simulink model "section_6_2_second_group"  (R2020a)
settings: Solver=ode45  StartTime=0.0  StopTime=50  RelTol=1e-5  EnableMultiTasking=on
(part 1 of 4)
settings Model: Creator=13018  LastModifiedBy=YW
settings DataIOCC: ReturnWorkspaceOutputs=off
settings OptimizationCC: LifeSpan=inf
settings DebuggingCC: SFUnexpectedBacktrackingDiag=warning  SFNoUnconditionalDefaultTransitionDiag=warning  ArithmeticOperatorsInVariantConditions=warning
settings SFSimCC: SimUseLocalCustomCode=off  CustomCodeUndefinedFunction=UseInterfaceOnly
settings RTWCC: RTWUseLocalCustomCode=off
settings CodeAppCC: StateflowObjectComments=on
settings GRTTargetCC: TargetLangStandard=C89/C90 (ANSI)
settings ConfigComp: CovMetricSettings=dw  CovHtmlReporting=on  CovSaveCumulativeToWorkspaceVar=on  CovSaveSingleToWorkspaceVar=on  CovExternalEMLEnable=off

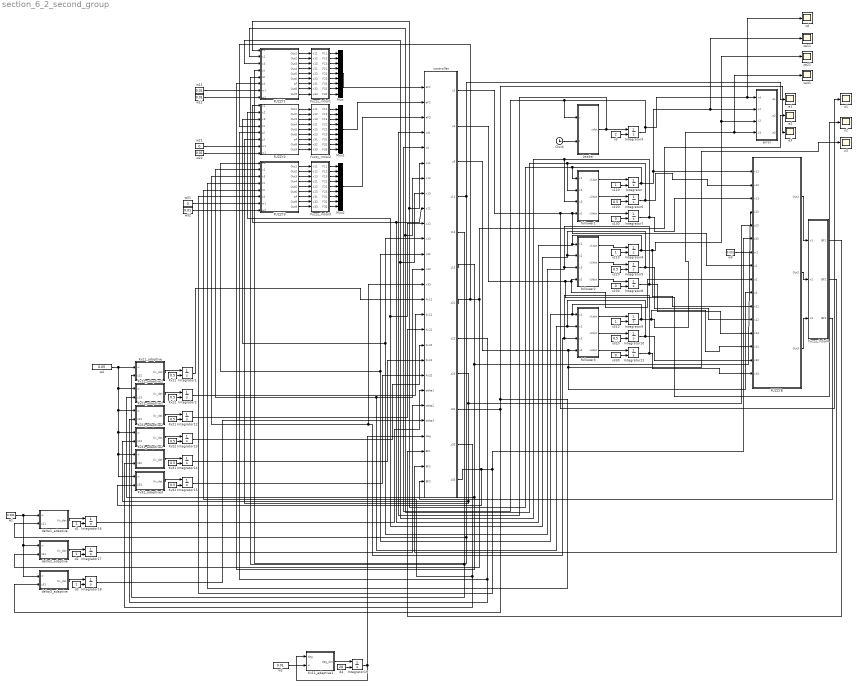
== system section_6_2_second_group ==
  Clock : Clock
  FUZZY1 : Subsystem
  FUZZY2 : Subsystem
  FUZZY3 : Subsystem
  FUZZYB : Subsystem
  Fuzzy_intial1 : MATLAB Function  TreatAsAtomicUnit=on
  Fuzzy_intial2 : MATLAB Function  TreatAsAtomicUnit=on
  Fuzzy_intial3 : MATLAB Function  TreatAsAtomicUnit=on
  Fuzzy_intial4 : MATLAB Function  TreatAsAtomicUnit=on
  Integrator{,1..19} (20 alike) : Integrator  InitialConditionSource=external
  Kv{11..12,21..22,31..32} (6 alike) : Constant  Value=0.5  VectorParams1D=off  SampleTime=-1
  Kv11_adaptive : MATLAB Function  TreatAsAtomicUnit=on
  Kv11_adaptive1 : MATLAB Function  TreatAsAtomicUnit=on
  Kv12_adaptive1 : MATLAB Function  TreatAsAtomicUnit=on
  Kv21_adaptive1 : MATLAB Function  TreatAsAtomicUnit=on
  Kv22_adaptive2 : MATLAB Function  TreatAsAtomicUnit=on
  Kv31_adaptive2 : MATLAB Function  TreatAsAtomicUnit=on
  Kv32_adaptive3 : MATLAB Function  TreatAsAtomicUnit=on
  Leader : MATLAB Function  TreatAsAtomicUnit=on
  Mux : Mux  Inputs=9
  Mux1 : Mux  Inputs=9
  Mux2 : Mux  Inputs=9
  controller : MATLAB Function  TreatAsAtomicUnit=on
  d1 : Constant  VectorParams1D=off  SampleTime=-1
  d2 : Constant  VectorParams1D=off  SampleTime=-1
  d3 : Constant  VectorParams1D=off  SampleTime=-1
  d4 : Constant  Value=20  VectorParams1D=off  SampleTime=-1
  delta1_adaptive : MATLAB Function  TreatAsAtomicUnit=on
  delta2_adaptive : MATLAB Function  TreatAsAtomicUnit=on
  delta3_adaptive : MATLAB Function  TreatAsAtomicUnit=on
  e1 : Scope
  e2 : Scope
  e3 : Scope
  error : MATLAB Function  TreatAsAtomicUnit=on
  follower1 : MATLAB Function  TreatAsAtomicUnit=on
  follower2 : MATLAB Function  TreatAsAtomicUnit=on
  follower3 : MATLAB Function  TreatAsAtomicUnit=on
  u1 : Scope
  u2 : Scope
  u3 : Scope
  w1 : Constant  Value=0.001  VectorParams1D=off  SampleTime=-1
  w{2,11..12,22,32} (5 alike) : Constant  Value=0.01  VectorParams1D=off  SampleTime=-1
  w21 : Constant  Value=0  VectorParams1D=off  SampleTime=-1
  w3 : Constant  Value=0.001  VectorParams1D=off  SampleTime=-1
  w31 : Constant  Value=0  VectorParams1D=off  SampleTime=-1
  w4 : Constant  Value=0.05  VectorParams1D=off  SampleTime=-1
  x0 : Constant  Value=2  VectorParams1D=off  SampleTime=-1
  x110 : Constant  VectorParams1D=off  SampleTime=-1
  x120 : Constant  Value=0.5  VectorParams1D=off  SampleTime=-1
  x130 : Constant  Value=0  VectorParams1D=off  SampleTime=-1
  x210 : Constant  VectorParams1D=off  SampleTime=-1
  x220 : Constant  Value=0.5  VectorParams1D=off  SampleTime=-1
  x230 : Constant  Value=0  VectorParams1D=off  SampleTime=-1
  x310 : Constant  VectorParams1D=off  SampleTime=-1
  x320 : Constant  Value=0.5  VectorParams1D=off  SampleTime=-1
  x330 : Constant  Value=0  VectorParams1D=off  SampleTime=-1
  xa11 : Scope
  xa21 : Scope
  xa31 : Scope
  xd : Scope
  wires:
  follower1/1(x1dot) -> Integrator/1
  Leader/1(xdot) -> controller/4(xdt), Integrator3/1
  x0/1 -> Integrator3/2
  follower1/2(x2dot) -> Integrator6/1
  follower1/3(x3dot) -> Integrator7/1
  x110/1 -> Integrator/2
  Integrator6/1 -> FUZZYB/2(x12), follower1/2(x2), FUZZY1/2(x2), controller/7(x12)
  Integrator7/1 -> FUZZYB/3(x13), FUZZY1/3(x3), controller/8(x13), follower1/3(x3)
  follower2/1(x1dot) -> Integrator4/1
  Integrator4/1 -> FUZZYB/11(x21), xa21/1, error/3(x2), FUZZY2/1(x1), controller/9(x21), follower2/1(x1)
  follower2/2(x2dot) -> Integrator5/1
  follower2/3(x3dot) -> Integrator8/1
  x210/1 -> Integrator4/2
  Integrator5/1 -> FUZZYB/12(x22), FUZZY2/2(x2), controller/10(x22), follower2/2(x2)
  Integrator8/1 -> FUZZYB/13(x23), FUZZY2/3(x3), controller/11(x23), follower2/3(x3)
  follower3/1(x1dot) -> Integrator9/1
  follower3/2(x2dot) -> Integrator10/1
  follower3/3(x3dot) -> Integrator11/1
  x310/1 -> Integrator9/2
  controller/1(u1) -> u1/1, FUZZYB/8(u1), follower1/4(u1)
  controller/2(u2) -> u2/1, FUZZYB/9(u2), follower2/4(u2)
  controller/3(u3) -> FUZZYB/10(u3), u3/1, follower3/4(u3)
  controller/5(z12) -> FUZZY1/5(z2), Kv11_adaptive/2(z12)
  controller/6(z13) -> FUZZYB/4(z13), FUZZY1/6(z3), Kv12_adaptive1/2(z13)
  controller/8(z22) -> FUZZY2/5(z2), Kv21_adaptive1/2(z22)
  controller/9(z23) -> FUZZYB/5(z23), FUZZY2/6(z3), Kv22_adaptive2/2(z23)
  controller/11(z32) -> FUZZY3/5(z2), Kv31_adaptive2/2(z32)
  controller/12(z33) -> FUZZYB/6(z33), FUZZY3/6(z3), Kv32_adaptive3/2(z33)
  Kv11_adaptive/1(Kv_dot) -> Integrator1/1
  Kv11/1 -> Integrator1/2
  Integrator1/1 -> controller/15(Kv11)
  Kv12_adaptive1/1(Kv_dot) -> Integrator2/1
  Kv12/1 -> Integrator2/2
  Kv21_adaptive1/1(Kv_dot) -> Integrator12/1
  Kv21/1 -> Integrator12/2
  Kv22_adaptive2/1(Kv_dot) -> Integrator13/1
  Kv22/1 -> Integrator13/2
  Kv31_adaptive2/1(Kv_dot) -> Integrator14/1
  Kv31/1 -> Integrator14/2
  Kv32_adaptive3/1(Kv_dot) -> Integrator15/1
  Kv32/1 -> Integrator15/2
  Integrator2/1 -> controller/16(Kv12)
  Integrator13/1 -> controller/18(Kv22)
  Integrator12/1 -> controller/17(Kv21)
  Integrator14/1 -> controller/19(Kv31)
  Integrator15/1 -> controller/20(Kv32)
  Clock/1 -> Leader/2(t)
  Mux/1 -> controller/1(aF1)
  Mux2/1 -> controller/3(aF3)
  Mux1/1 -> controller/2(aF2)
  w11/1 -> FUZZY1/7(w1)
  w12/1 -> FUZZY1/8(w2)
  w21/1 -> FUZZY2/7(w1)
  w22/1 -> FUZZY2/8(w2)
  w32/1 -> FUZZY3/8(w2)
  w31/1 -> FUZZY3/7(w1)
  delta1_adaptive/1(Kv_dot) -> Integrator16/1
  d1/1 -> Integrator16/2
  delta2_adaptive/1(Kv_dot) -> Integrator17/1
  d2/1 -> Integrator17/2
  delta3_adaptive/1(Kv_dot) -> Integrator18/1
  d3/1 -> Integrator18/2
  w1/1 -> delta3_adaptive/1(w), delta2_adaptive/1(w), delta1_adaptive/1(w)
  Integrator16/1 -> controller/21(delta1)
  Integrator17/1 -> controller/22(delta2)
  Integrator18/1 -> controller/23(delta3)
  FUZZY1/1(Out1) -> Fuzzy_intial1/1(x11)
  FUZZY1/2(Out2) -> Fuzzy_intial1/2(x12)
  FUZZY1/3(Out3) -> Fuzzy_intial1/3(x13)
  FUZZY1/4(Out4) -> Fuzzy_intial1/4(x21)
  FUZZY1/5(Out5) -> Fuzzy_intial1/5(x22)
  FUZZY1/6(Out6) -> Fuzzy_intial1/6(x23)
  FUZZY1/7(aF) -> Fuzzy_intial1/7(x31)
  FUZZY1/8(Out8) -> Fuzzy_intial1/8(x32)
  FUZZY1/9(Out9) -> Fuzzy_intial1/9(x33)
  Fuzzy_intial1/1(F11) -> Mux/1
  Fuzzy_intial1/2(F12) -> Mux/2
  Fuzzy_intial1/3(F13) -> Mux/3
  Fuzzy_intial1/4(F21) -> Mux/4
  Fuzzy_intial1/5(F22) -> Mux/5
  Fuzzy_intial1/6(F23) -> Mux/6
  Fuzzy_intial1/7(F31) -> Mux/7
  Fuzzy_intial1/8(F32) -> Mux/8
  Fuzzy_intial1/9(F33) -> Mux/9
  Fuzzy_intial2/1(F11) -> Mux1/1
  Fuzzy_intial2/2(F12) -> Mux1/2
  Fuzzy_intial2/3(F13) -> Mux1/3
  Fuzzy_intial2/4(F21) -> Mux1/4
  Fuzzy_intial2/5(F22) -> Mux1/5
  Fuzzy_intial2/6(F23) -> Mux1/6
  Fuzzy_intial2/7(F31) -> Mux1/7
  Fuzzy_intial2/8(F32) -> Mux1/8
  Fuzzy_intial2/9(F33) -> Mux1/9
  FUZZY2/1(Out1) -> Fuzzy_intial2/1(x11)
  FUZZY2/2(Out2) -> Fuzzy_intial2/2(x12)
  FUZZY2/3(Out3) -> Fuzzy_intial2/3(x13)
  FUZZY2/4(Out4) -> Fuzzy_intial2/4(x21)
  FUZZY2/5(Out5) -> Fuzzy_intial2/5(x22)
  FUZZY2/6(Out6) -> Fuzzy_intial2/6(x23)
  FUZZY2/7(aF) -> Fuzzy_intial2/7(x31)
  FUZZY2/8(Out8) -> Fuzzy_intial2/8(x32)
  FUZZY2/9(Out9) -> Fuzzy_intial2/9(x33)
  Fuzzy_intial3/1(F11) -> Mux2/1
  Fuzzy_intial3/2(F12) -> Mux2/2
  Fuzzy_intial3/3(F13) -> Mux2/3
  Fuzzy_intial3/4(F21) -> Mux2/4
  Fuzzy_intial3/5(F22) -> Mux2/5
  Fuzzy_intial3/6(F23) -> Mux2/6
  Fuzzy_intial3/7(F31) -> Mux2/7
  Fuzzy_intial3/8(F32) -> Mux2/8
  Fuzzy_intial3/9(F33) -> Mux2/9
  FUZZY3/1(Out1) -> Fuzzy_intial3/1(x11)
  FUZZY3/2(Out2) -> Fuzzy_intial3/2(x12)
  FUZZY3/3(Out3) -> Fuzzy_intial3/3(x13)
  FUZZY3/4(Out4) -> Fuzzy_intial3/4(x21)
  FUZZY3/5(Out5) -> Fuzzy_intial3/5(x22)
  FUZZY3/6(Out6) -> Fuzzy_intial3/6(x23)
  FUZZY3/7(aF) -> Fuzzy_intial3/7(x31)
  FUZZY3/8(Out8) -> Fuzzy_intial3/8(x32)
  FUZZY3/9(Out9) -> Fuzzy_intial3/9(x33)
  w4/1 -> Kv32_adaptive3/1(w), Kv31_adaptive2/1(w), Kv22_adaptive2/1(w), Kv21_adaptive1/1(w), Kv12_adaptive1/1(w), Kv11_adaptive/1(w)
  Kv11_adaptive1/1(dag_dot) -> Integrator19/1
  d4/1 -> Integrator19/2
  Integrator19/1 -> controller/24(dag), Kv11_adaptive1/1(dag)
  w2/1 -> Kv11_adaptive1/2(w)
  Integrator10/1 -> FUZZYB/15(x32), follower3/2(x2), FUZZY3/2(x2), controller/13(x32)
  Integrator11/1 -> FUZZYB/16(x33), FUZZY3/3(x3), controller/14(x33), follower3/3(x3)
  FUZZYB/1(Out1) -> Fuzzy_intial4/1(x1)
  FUZZYB/2(Out2) -> Fuzzy_intial4/2(x2)
  FUZZYB/3(Out3) -> Fuzzy_intial4/3(x3)
  Fuzzy_intial4/1(BF1) -> controller/25(BF1)
  Fuzzy_intial4/2(BF2) -> controller/26(BF2)
  Fuzzy_intial4/3(BF3) -> controller/27(BF3)
  w3/1 -> FUZZYB/7(w1)
  controller/4(z11) -> FUZZY1/4(z1), delta1_adaptive/2(z11), e1/1
  controller/7(z21) -> FUZZY2/4(z1), delta2_adaptive/2(z21), e2/1
  controller/10(z31) -> FUZZY3/4(z1), e3/1, delta3_adaptive/2(z31)
  x120/1 -> Integrator6/2
  x130/1 -> Integrator7/2
  x220/1 -> Integrator5/2
  x230/1 -> Integrator8/2
  x320/1 -> Integrator10/2
  x330/1 -> Integrator11/2
  Integrator3/1 -> xd/1, error/1(xd), Leader/1(x), controller/5(xd)
  Integrator/1 -> FUZZYB/1(x11), xa11/1, error/2(x1), follower1/1(x1), FUZZY1/1(x1), controller/6(x11)
  Integrator9/1 -> FUZZYB/14(x31), xa31/1, error/4(x3), FUZZY3/1(x1), controller/12(x31), follower3/1(x1)

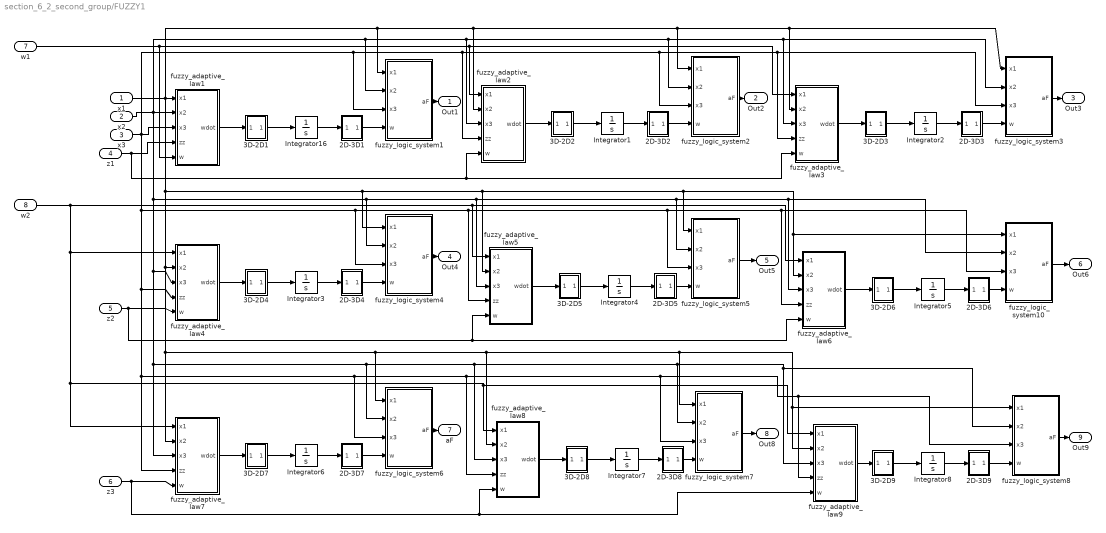
== system section_6_2_second_group/FUZZY1 ==
  x1 : Inport
  x2 : Inport  Port=2
  x3 : Inport  Port=3
  z1 : Inport  Port=4
  z2 : Inport  Port=5
  z3 : Inport  Port=6
  w1 : Inport  Port=7
  w2 : Inport  Port=8
  2D-3D1 : MATLAB Function  TreatAsAtomicUnit=on
  2D-3D2 : MATLAB Function  TreatAsAtomicUnit=on
  2D-3D3 : MATLAB Function  TreatAsAtomicUnit=on
  2D-3D4 : MATLAB Function  TreatAsAtomicUnit=on
  2D-3D5 : MATLAB Function  TreatAsAtomicUnit=on
  2D-3D6 : MATLAB Function  TreatAsAtomicUnit=on
  2D-3D7 : MATLAB Function  TreatAsAtomicUnit=on
  2D-3D8 : MATLAB Function  TreatAsAtomicUnit=on
  2D-3D9 : MATLAB Function  TreatAsAtomicUnit=on
  3D-2D1 : MATLAB Function  TreatAsAtomicUnit=on
  3D-2D2 : MATLAB Function  TreatAsAtomicUnit=on
  3D-2D3 : MATLAB Function  TreatAsAtomicUnit=on
  3D-2D4 : MATLAB Function  TreatAsAtomicUnit=on
  3D-2D5 : MATLAB Function  TreatAsAtomicUnit=on
  3D-2D6 : MATLAB Function  TreatAsAtomicUnit=on
  3D-2D7 : MATLAB Function  TreatAsAtomicUnit=on
  3D-2D8 : MATLAB Function  TreatAsAtomicUnit=on
  3D-2D9 : MATLAB Function  TreatAsAtomicUnit=on
  Integrator{1..8,16} (9 alike) : Integrator
  fuzzy_adaptive_law1 : MATLAB Function  TreatAsAtomicUnit=on
  fuzzy_adaptive_law2 : MATLAB Function  TreatAsAtomicUnit=on
  fuzzy_adaptive_law3 : MATLAB Function  TreatAsAtomicUnit=on
  fuzzy_adaptive_law4 : MATLAB Function  TreatAsAtomicUnit=on
  fuzzy_adaptive_law5 : MATLAB Function  TreatAsAtomicUnit=on
  fuzzy_adaptive_law6 : MATLAB Function  TreatAsAtomicUnit=on
  fuzzy_adaptive_law7 : MATLAB Function  TreatAsAtomicUnit=on
  fuzzy_adaptive_law8 : MATLAB Function  TreatAsAtomicUnit=on
  fuzzy_adaptive_law9 : MATLAB Function  TreatAsAtomicUnit=on
  fuzzy_logic_system1 : MATLAB Function  TreatAsAtomicUnit=on
  fuzzy_logic_system10 : MATLAB Function  TreatAsAtomicUnit=on
  fuzzy_logic_system2 : MATLAB Function  TreatAsAtomicUnit=on
  fuzzy_logic_system3 : MATLAB Function  TreatAsAtomicUnit=on
  fuzzy_logic_system4 : MATLAB Function  TreatAsAtomicUnit=on
  fuzzy_logic_system5 : MATLAB Function  TreatAsAtomicUnit=on
  fuzzy_logic_system6 : MATLAB Function  TreatAsAtomicUnit=on
  fuzzy_logic_system7 : MATLAB Function  TreatAsAtomicUnit=on
  fuzzy_logic_system8 : MATLAB Function  TreatAsAtomicUnit=on
  Out1 : Outport
  Out2 : Outport  Port=2
  Out3 : Outport  Port=3
  Out4 : Outport  Port=4
  Out5 : Outport  Port=5
  Out6 : Outport  Port=6
  aF : Outport  Port=7
  Out8 : Outport  Port=8
  Out9 : Outport  Port=9
  wires:
  3D-2D1/1(y) -> Integrator16/1
  fuzzy_adaptive_law1/1(wdot) -> 3D-2D1/1(x)
  Integrator16/1 -> 2D-3D1/1(x)
  2D-3D1/1(y) -> fuzzy_logic_system1/4(w)
  3D-2D2/1(y) -> Integrator1/1
  fuzzy_adaptive_law2/1(wdot) -> 3D-2D2/1(x)
  Integrator1/1 -> 2D-3D2/1(x)
  2D-3D2/1(y) -> fuzzy_logic_system2/4(w)
  3D-2D3/1(y) -> Integrator2/1
  fuzzy_adaptive_law3/1(wdot) -> 3D-2D3/1(x)
  Integrator2/1 -> 2D-3D3/1(x)
  2D-3D3/1(y) -> fuzzy_logic_system3/4(w)
  x1/1 -> fuzzy_adaptive_law4/2(x2), fuzzy_adaptive_law7/2(x2), fuzzy_logic_system6/1(x1), fuzzy_adaptive_law8/2(x2), fuzzy_adaptive_law9/2(x2), fuzzy_logic_system8/1(x1), fuzzy_logic_system7/1(x1), fuzzy_adaptive_law5/2(x2), fuzzy_logic_system5/1(x1), fuzzy_adaptive_law6/2(x2), fuzzy_logic_system10/1(x1), fuzzy_logic_system4/1(x1), fuzzy_adaptive_law1/1(x1), fuzzy_logic_system1/1(x1), fuzzy_adaptive_law2/2(x2), fuzzy_logic_system2/1(x1), fuzzy_adaptive_law3/2(x2), fuzzy_logic_system3/1(x1)
  x2/1 -> fuzzy_logic_system4/2(x2), fuzzy_adaptive_law5/3(x3), fuzzy_logic_system5/2(x2), fuzzy_adaptive_law6/3(x3), fuzzy_logic_system10/2(x2), fuzzy_adaptive_law4/3(x3), fuzzy_adaptive_law7/3(x3), fuzzy_logic_system6/2(x2), fuzzy_adaptive_law8/3(x3), fuzzy_logic_system7/2(x2), fuzzy_adaptive_law9/3(x3), fuzzy_logic_system8/2(x2), fuzzy_adaptive_law1/2(x2), fuzzy_logic_system1/2(x2), fuzzy_adaptive_law2/3(x3), fuzzy_logic_system2/2(x2), fuzzy_adaptive_law3/3(x3), fuzzy_logic_system3/2(x2)
  x3/1 -> fuzzy_adaptive_law1/3(x3), fuzzy_logic_system4/3(x3), fuzzy_adaptive_law5/4(zz), fuzzy_logic_system5/3(x3), fuzzy_adaptive_law6/4(zz), fuzzy_logic_system10/3(x3), fuzzy_adaptive_law4/4(zz), fuzzy_adaptive_law7/4(zz), fuzzy_logic_system6/3(x3), fuzzy_adaptive_law8/4(zz), fuzzy_logic_system7/3(x3), fuzzy_adaptive_law9/4(zz), fuzzy_logic_system8/3(x3), fuzzy_logic_system1/3(x3), fuzzy_logic_system2/3(x3), fuzzy_adaptive_law3/4(zz), fuzzy_logic_system3/3(x3), fuzzy_adaptive_law2/4(zz)
  z1/1 -> fuzzy_adaptive_law1/4(zz), fuzzy_adaptive_law3/5(w), fuzzy_adaptive_law2/5(w)
  3D-2D4/1(y) -> Integrator3/1
  fuzzy_adaptive_law4/1(wdot) -> 3D-2D4/1(x)
  Integrator3/1 -> 2D-3D4/1(x)
  2D-3D4/1(y) -> fuzzy_logic_system4/4(w)
  3D-2D5/1(y) -> Integrator4/1
  fuzzy_adaptive_law5/1(wdot) -> 3D-2D5/1(x)
  Integrator4/1 -> 2D-3D5/1(x)
  2D-3D5/1(y) -> fuzzy_logic_system5/4(w)
  3D-2D6/1(y) -> Integrator5/1
  fuzzy_adaptive_law6/1(wdot) -> 3D-2D6/1(x)
  Integrator5/1 -> 2D-3D6/1(x)
  2D-3D6/1(y) -> fuzzy_logic_system10/4(w)
  3D-2D7/1(y) -> Integrator6/1
  fuzzy_adaptive_law7/1(wdot) -> 3D-2D7/1(x)
  Integrator6/1 -> 2D-3D7/1(x)
  2D-3D7/1(y) -> fuzzy_logic_system6/4(w)
  3D-2D8/1(y) -> Integrator7/1
  fuzzy_adaptive_law8/1(wdot) -> 3D-2D8/1(x)
  Integrator7/1 -> 2D-3D8/1(x)
  2D-3D8/1(y) -> fuzzy_logic_system7/4(w)
  3D-2D9/1(y) -> Integrator8/1
  fuzzy_adaptive_law9/1(wdot) -> 3D-2D9/1(x)
  Integrator8/1 -> 2D-3D9/1(x)
  2D-3D9/1(y) -> fuzzy_logic_system8/4(w)
  z2/1 -> fuzzy_adaptive_law4/5(w), fuzzy_adaptive_law5/5(w), fuzzy_adaptive_law6/5(w)
  z3/1 -> fuzzy_adaptive_law7/5(w), fuzzy_adaptive_law8/5(w), fuzzy_adaptive_law9/5(w)
  fuzzy_logic_system1/1(aF) -> Out1/1
  fuzzy_logic_system2/1(aF) -> Out2/1
  fuzzy_logic_system3/1(aF) -> Out3/1
  fuzzy_logic_system4/1(aF) -> Out4/1
  fuzzy_logic_system5/1(aF) -> Out5/1
  fuzzy_logic_system10/1(aF) -> Out6/1
  fuzzy_logic_system6/1(aF) -> aF/1
  fuzzy_logic_system7/1(aF) -> Out8/1
  fuzzy_logic_system8/1(aF) -> Out9/1
  w2/1 -> fuzzy_adaptive_law4/1(x1), fuzzy_adaptive_law7/1(x1), fuzzy_adaptive_law8/1(x1), fuzzy_adaptive_law9/1(x1), fuzzy_adaptive_law5/1(x1), fuzzy_adaptive_law6/1(x1)
  w1/1 -> fuzzy_adaptive_law1/5(w), fuzzy_adaptive_law3/1(x1), fuzzy_adaptive_law2/1(x1)

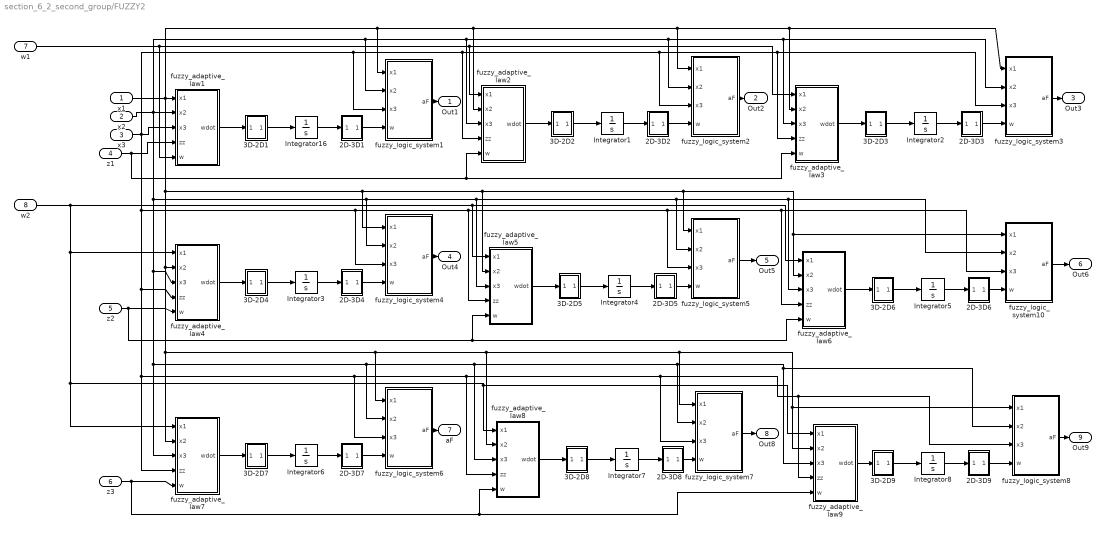
== system section_6_2_second_group/FUZZY2 ==
  x1 : Inport
  x2 : Inport  Port=2
  x3 : Inport  Port=3
  z1 : Inport  Port=4
  z2 : Inport  Port=5
  z3 : Inport  Port=6
  w1 : Inport  Port=7
  w2 : Inport  Port=8
  2D-3D1 : MATLAB Function  TreatAsAtomicUnit=on
  2D-3D2 : MATLAB Function  TreatAsAtomicUnit=on
  2D-3D3 : MATLAB Function  TreatAsAtomicUnit=on
  2D-3D4 : MATLAB Function  TreatAsAtomicUnit=on
  2D-3D5 : MATLAB Function  TreatAsAtomicUnit=on
  2D-3D6 : MATLAB Function  TreatAsAtomicUnit=on
  2D-3D7 : MATLAB Function  TreatAsAtomicUnit=on
  2D-3D8 : MATLAB Function  TreatAsAtomicUnit=on
  2D-3D9 : MATLAB Function  TreatAsAtomicUnit=on
  3D-2D1 : MATLAB Function  TreatAsAtomicUnit=on
  3D-2D2 : MATLAB Function  TreatAsAtomicUnit=on
  3D-2D3 : MATLAB Function  TreatAsAtomicUnit=on
  3D-2D4 : MATLAB Function  TreatAsAtomicUnit=on
  3D-2D5 : MATLAB Function  TreatAsAtomicUnit=on
  3D-2D6 : MATLAB Function  TreatAsAtomicUnit=on
  3D-2D7 : MATLAB Function  TreatAsAtomicUnit=on
  3D-2D8 : MATLAB Function  TreatAsAtomicUnit=on
  3D-2D9 : MATLAB Function  TreatAsAtomicUnit=on
  Integrator{1..8,16} (9 alike) : Integrator
  fuzzy_adaptive_law1 : MATLAB Function  TreatAsAtomicUnit=on
  fuzzy_adaptive_law2 : MATLAB Function  TreatAsAtomicUnit=on
  fuzzy_adaptive_law3 : MATLAB Function  TreatAsAtomicUnit=on
  fuzzy_adaptive_law4 : MATLAB Function  TreatAsAtomicUnit=on
  fuzzy_adaptive_law5 : MATLAB Function  TreatAsAtomicUnit=on
  fuzzy_adaptive_law6 : MATLAB Function  TreatAsAtomicUnit=on
  fuzzy_adaptive_law7 : MATLAB Function  TreatAsAtomicUnit=on
  fuzzy_adaptive_law8 : MATLAB Function  TreatAsAtomicUnit=on
  fuzzy_adaptive_law9 : MATLAB Function  TreatAsAtomicUnit=on
  fuzzy_logic_system1 : MATLAB Function  TreatAsAtomicUnit=on
  fuzzy_logic_system10 : MATLAB Function  TreatAsAtomicUnit=on
  fuzzy_logic_system2 : MATLAB Function  TreatAsAtomicUnit=on
  fuzzy_logic_system3 : MATLAB Function  TreatAsAtomicUnit=on
  fuzzy_logic_system4 : MATLAB Function  TreatAsAtomicUnit=on
  fuzzy_logic_system5 : MATLAB Function  TreatAsAtomicUnit=on
  fuzzy_logic_system6 : MATLAB Function  TreatAsAtomicUnit=on
  fuzzy_logic_system7 : MATLAB Function  TreatAsAtomicUnit=on
  fuzzy_logic_system8 : MATLAB Function  TreatAsAtomicUnit=on
  Out1 : Outport
  Out2 : Outport  Port=2
  Out3 : Outport  Port=3
  Out4 : Outport  Port=4
  Out5 : Outport  Port=5
  Out6 : Outport  Port=6
  aF : Outport  Port=7
  Out8 : Outport  Port=8
  Out9 : Outport  Port=9
  wires:
  3D-2D1/1(y) -> Integrator16/1
  fuzzy_adaptive_law1/1(wdot) -> 3D-2D1/1(x)
  Integrator16/1 -> 2D-3D1/1(x)
  2D-3D1/1(y) -> fuzzy_logic_system1/4(w)
  3D-2D2/1(y) -> Integrator1/1
  fuzzy_adaptive_law2/1(wdot) -> 3D-2D2/1(x)
  Integrator1/1 -> 2D-3D2/1(x)
  2D-3D2/1(y) -> fuzzy_logic_system2/4(w)
  3D-2D3/1(y) -> Integrator2/1
  fuzzy_adaptive_law3/1(wdot) -> 3D-2D3/1(x)
  Integrator2/1 -> 2D-3D3/1(x)
  2D-3D3/1(y) -> fuzzy_logic_system3/4(w)
  x1/1 -> fuzzy_adaptive_law4/2(x2), fuzzy_adaptive_law7/2(x2), fuzzy_logic_system6/1(x1), fuzzy_adaptive_law8/2(x2), fuzzy_adaptive_law9/2(x2), fuzzy_logic_system8/1(x1), fuzzy_logic_system7/1(x1), fuzzy_adaptive_law5/2(x2), fuzzy_logic_system5/1(x1), fuzzy_adaptive_law6/2(x2), fuzzy_logic_system10/1(x1), fuzzy_logic_system4/1(x1), fuzzy_adaptive_law1/1(x1), fuzzy_logic_system1/1(x1), fuzzy_adaptive_law2/2(x2), fuzzy_logic_system2/1(x1), fuzzy_adaptive_law3/2(x2), fuzzy_logic_system3/1(x1)
  x2/1 -> fuzzy_logic_system4/2(x2), fuzzy_adaptive_law5/3(x3), fuzzy_logic_system5/2(x2), fuzzy_adaptive_law6/3(x3), fuzzy_logic_system10/2(x2), fuzzy_adaptive_law4/3(x3), fuzzy_adaptive_law7/3(x3), fuzzy_logic_system6/2(x2), fuzzy_adaptive_law8/3(x3), fuzzy_logic_system7/2(x2), fuzzy_adaptive_law9/3(x3), fuzzy_logic_system8/2(x2), fuzzy_adaptive_law1/2(x2), fuzzy_logic_system1/2(x2), fuzzy_adaptive_law2/3(x3), fuzzy_logic_system2/2(x2), fuzzy_adaptive_law3/3(x3), fuzzy_logic_system3/2(x2)
  x3/1 -> fuzzy_adaptive_law1/3(x3), fuzzy_logic_system4/3(x3), fuzzy_adaptive_law5/4(zz), fuzzy_logic_system5/3(x3), fuzzy_adaptive_law6/4(zz), fuzzy_logic_system10/3(x3), fuzzy_adaptive_law4/4(zz), fuzzy_adaptive_law7/4(zz), fuzzy_logic_system6/3(x3), fuzzy_adaptive_law8/4(zz), fuzzy_logic_system7/3(x3), fuzzy_adaptive_law9/4(zz), fuzzy_logic_system8/3(x3), fuzzy_logic_system1/3(x3), fuzzy_logic_system2/3(x3), fuzzy_adaptive_law3/4(zz), fuzzy_logic_system3/3(x3), fuzzy_adaptive_law2/4(zz)
  z1/1 -> fuzzy_adaptive_law1/4(zz), fuzzy_adaptive_law3/5(w), fuzzy_adaptive_law2/5(w)
  3D-2D4/1(y) -> Integrator3/1
  fuzzy_adaptive_law4/1(wdot) -> 3D-2D4/1(x)
  Integrator3/1 -> 2D-3D4/1(x)
  2D-3D4/1(y) -> fuzzy_logic_system4/4(w)
  3D-2D5/1(y) -> Integrator4/1
  fuzzy_adaptive_law5/1(wdot) -> 3D-2D5/1(x)
  Integrator4/1 -> 2D-3D5/1(x)
  2D-3D5/1(y) -> fuzzy_logic_system5/4(w)
  3D-2D6/1(y) -> Integrator5/1
  fuzzy_adaptive_law6/1(wdot) -> 3D-2D6/1(x)
  Integrator5/1 -> 2D-3D6/1(x)
  2D-3D6/1(y) -> fuzzy_logic_system10/4(w)
  3D-2D7/1(y) -> Integrator6/1
  fuzzy_adaptive_law7/1(wdot) -> 3D-2D7/1(x)
  Integrator6/1 -> 2D-3D7/1(x)
  2D-3D7/1(y) -> fuzzy_logic_system6/4(w)
  3D-2D8/1(y) -> Integrator7/1
  fuzzy_adaptive_law8/1(wdot) -> 3D-2D8/1(x)
  Integrator7/1 -> 2D-3D8/1(x)
  2D-3D8/1(y) -> fuzzy_logic_system7/4(w)
  3D-2D9/1(y) -> Integrator8/1
  fuzzy_adaptive_law9/1(wdot) -> 3D-2D9/1(x)
  Integrator8/1 -> 2D-3D9/1(x)
  2D-3D9/1(y) -> fuzzy_logic_system8/4(w)
  z2/1 -> fuzzy_adaptive_law4/5(w), fuzzy_adaptive_law5/5(w), fuzzy_adaptive_law6/5(w)
  z3/1 -> fuzzy_adaptive_law7/5(w), fuzzy_adaptive_law8/5(w), fuzzy_adaptive_law9/5(w)
  fuzzy_logic_system1/1(aF) -> Out1/1
  fuzzy_logic_system2/1(aF) -> Out2/1
  fuzzy_logic_system3/1(aF) -> Out3/1
  fuzzy_logic_system4/1(aF) -> Out4/1
  fuzzy_logic_system5/1(aF) -> Out5/1
  fuzzy_logic_system10/1(aF) -> Out6/1
  fuzzy_logic_system6/1(aF) -> aF/1
  fuzzy_logic_system7/1(aF) -> Out8/1
  fuzzy_logic_system8/1(aF) -> Out9/1
  w2/1 -> fuzzy_adaptive_law4/1(x1), fuzzy_adaptive_law7/1(x1), fuzzy_adaptive_law8/1(x1), fuzzy_adaptive_law9/1(x1), fuzzy_adaptive_law5/1(x1), fuzzy_adaptive_law6/1(x1)
  w1/1 -> fuzzy_adaptive_law1/5(w), fuzzy_adaptive_law3/1(x1), fuzzy_adaptive_law2/1(x1)

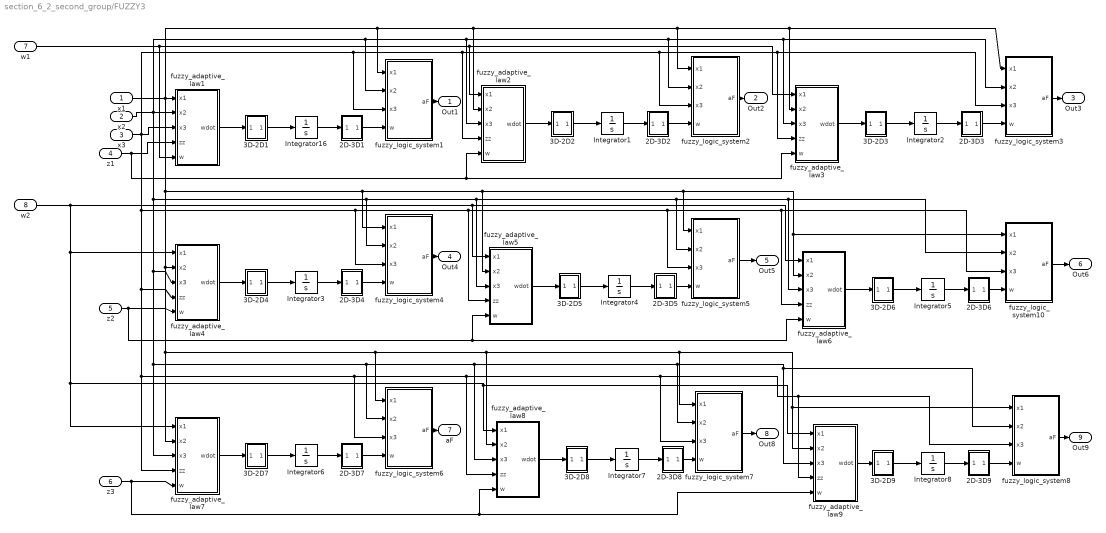
== system section_6_2_second_group/FUZZY3 ==
  x1 : Inport
  x2 : Inport  Port=2
  x3 : Inport  Port=3
  z1 : Inport  Port=4
  z2 : Inport  Port=5
  z3 : Inport  Port=6
  w1 : Inport  Port=7
  w2 : Inport  Port=8
  2D-3D1 : MATLAB Function  TreatAsAtomicUnit=on
  2D-3D2 : MATLAB Function  TreatAsAtomicUnit=on
  2D-3D3 : MATLAB Function  TreatAsAtomicUnit=on
  2D-3D4 : MATLAB Function  TreatAsAtomicUnit=on
  2D-3D5 : MATLAB Function  TreatAsAtomicUnit=on
  2D-3D6 : MATLAB Function  TreatAsAtomicUnit=on
  2D-3D7 : MATLAB Function  TreatAsAtomicUnit=on
  2D-3D8 : MATLAB Function  TreatAsAtomicUnit=on
  2D-3D9 : MATLAB Function  TreatAsAtomicUnit=on
  3D-2D1 : MATLAB Function  TreatAsAtomicUnit=on
  3D-2D2 : MATLAB Function  TreatAsAtomicUnit=on
  3D-2D3 : MATLAB Function  TreatAsAtomicUnit=on
  3D-2D4 : MATLAB Function  TreatAsAtomicUnit=on
  3D-2D5 : MATLAB Function  TreatAsAtomicUnit=on
  3D-2D6 : MATLAB Function  TreatAsAtomicUnit=on
  3D-2D7 : MATLAB Function  TreatAsAtomicUnit=on
  3D-2D8 : MATLAB Function  TreatAsAtomicUnit=on
  3D-2D9 : MATLAB Function  TreatAsAtomicUnit=on
  Integrator{1..8,16} (9 alike) : Integrator
  fuzzy_adaptive_law1 : MATLAB Function  TreatAsAtomicUnit=on
  fuzzy_adaptive_law2 : MATLAB Function  TreatAsAtomicUnit=on
  fuzzy_adaptive_law3 : MATLAB Function  TreatAsAtomicUnit=on
  fuzzy_adaptive_law4 : MATLAB Function  TreatAsAtomicUnit=on
  fuzzy_adaptive_law5 : MATLAB Function  TreatAsAtomicUnit=on
  fuzzy_adaptive_law6 : MATLAB Function  TreatAsAtomicUnit=on
  fuzzy_adaptive_law7 : MATLAB Function  TreatAsAtomicUnit=on
  fuzzy_adaptive_law8 : MATLAB Function  TreatAsAtomicUnit=on
  fuzzy_adaptive_law9 : MATLAB Function  TreatAsAtomicUnit=on
  fuzzy_logic_system1 : MATLAB Function  TreatAsAtomicUnit=on
  fuzzy_logic_system10 : MATLAB Function  TreatAsAtomicUnit=on
  fuzzy_logic_system2 : MATLAB Function  TreatAsAtomicUnit=on
  fuzzy_logic_system3 : MATLAB Function  TreatAsAtomicUnit=on
  fuzzy_logic_system4 : MATLAB Function  TreatAsAtomicUnit=on
  fuzzy_logic_system5 : MATLAB Function  TreatAsAtomicUnit=on
  fuzzy_logic_system6 : MATLAB Function  TreatAsAtomicUnit=on
  fuzzy_logic_system7 : MATLAB Function  TreatAsAtomicUnit=on
  fuzzy_logic_system8 : MATLAB Function  TreatAsAtomicUnit=on
  Out1 : Outport
  Out2 : Outport  Port=2
  Out3 : Outport  Port=3
  Out4 : Outport  Port=4
  Out5 : Outport  Port=5
  Out6 : Outport  Port=6
  aF : Outport  Port=7
  Out8 : Outport  Port=8
  Out9 : Outport  Port=9
  wires:
  3D-2D1/1(y) -> Integrator16/1
  fuzzy_adaptive_law1/1(wdot) -> 3D-2D1/1(x)
  Integrator16/1 -> 2D-3D1/1(x)
  2D-3D1/1(y) -> fuzzy_logic_system1/4(w)
  3D-2D2/1(y) -> Integrator1/1
  fuzzy_adaptive_law2/1(wdot) -> 3D-2D2/1(x)
  Integrator1/1 -> 2D-3D2/1(x)
  2D-3D2/1(y) -> fuzzy_logic_system2/4(w)
  3D-2D3/1(y) -> Integrator2/1
  fuzzy_adaptive_law3/1(wdot) -> 3D-2D3/1(x)
  Integrator2/1 -> 2D-3D3/1(x)
  2D-3D3/1(y) -> fuzzy_logic_system3/4(w)
  x1/1 -> fuzzy_adaptive_law4/2(x2), fuzzy_adaptive_law7/2(x2), fuzzy_logic_system6/1(x1), fuzzy_adaptive_law8/2(x2), fuzzy_adaptive_law9/2(x2), fuzzy_logic_system8/1(x1), fuzzy_logic_system7/1(x1), fuzzy_adaptive_law5/2(x2), fuzzy_logic_system5/1(x1), fuzzy_adaptive_law6/2(x2), fuzzy_logic_system10/1(x1), fuzzy_logic_system4/1(x1), fuzzy_adaptive_law1/1(x1), fuzzy_logic_system1/1(x1), fuzzy_adaptive_law2/2(x2), fuzzy_logic_system2/1(x1), fuzzy_adaptive_law3/2(x2), fuzzy_logic_system3/1(x1)
  x2/1 -> fuzzy_logic_system4/2(x2), fuzzy_adaptive_law5/3(x3), fuzzy_logic_system5/2(x2), fuzzy_adaptive_law6/3(x3), fuzzy_logic_system10/2(x2), fuzzy_adaptive_law4/3(x3), fuzzy_adaptive_law7/3(x3), fuzzy_logic_system6/2(x2), fuzzy_adaptive_law8/3(x3), fuzzy_logic_system7/2(x2), fuzzy_adaptive_law9/3(x3), fuzzy_logic_system8/2(x2), fuzzy_adaptive_law1/2(x2), fuzzy_logic_system1/2(x2), fuzzy_adaptive_law2/3(x3), fuzzy_logic_system2/2(x2), fuzzy_adaptive_law3/3(x3), fuzzy_logic_system3/2(x2)
  x3/1 -> fuzzy_adaptive_law1/3(x3), fuzzy_logic_system4/3(x3), fuzzy_adaptive_law5/4(zz), fuzzy_logic_system5/3(x3), fuzzy_adaptive_law6/4(zz), fuzzy_logic_system10/3(x3), fuzzy_adaptive_law4/4(zz), fuzzy_adaptive_law7/4(zz), fuzzy_logic_system6/3(x3), fuzzy_adaptive_law8/4(zz), fuzzy_logic_system7/3(x3), fuzzy_adaptive_law9/4(zz), fuzzy_logic_system8/3(x3), fuzzy_logic_system1/3(x3), fuzzy_logic_system2/3(x3), fuzzy_adaptive_law3/4(zz), fuzzy_logic_system3/3(x3), fuzzy_adaptive_law2/4(zz)
  z1/1 -> fuzzy_adaptive_law1/4(zz), fuzzy_adaptive_law3/5(w), fuzzy_adaptive_law2/5(w)
  3D-2D4/1(y) -> Integrator3/1
  fuzzy_adaptive_law4/1(wdot) -> 3D-2D4/1(x)
  Integrator3/1 -> 2D-3D4/1(x)
  2D-3D4/1(y) -> fuzzy_logic_system4/4(w)
  3D-2D5/1(y) -> Integrator4/1
  fuzzy_adaptive_law5/1(wdot) -> 3D-2D5/1(x)
  Integrator4/1 -> 2D-3D5/1(x)
  2D-3D5/1(y) -> fuzzy_logic_system5/4(w)
  3D-2D6/1(y) -> Integrator5/1
  fuzzy_adaptive_law6/1(wdot) -> 3D-2D6/1(x)
  Integrator5/1 -> 2D-3D6/1(x)
  2D-3D6/1(y) -> fuzzy_logic_system10/4(w)
  3D-2D7/1(y) -> Integrator6/1
  fuzzy_adaptive_law7/1(wdot) -> 3D-2D7/1(x)
  Integrator6/1 -> 2D-3D7/1(x)
  2D-3D7/1(y) -> fuzzy_logic_system6/4(w)
  3D-2D8/1(y) -> Integrator7/1
  fuzzy_adaptive_law8/1(wdot) -> 3D-2D8/1(x)
  Integrator7/1 -> 2D-3D8/1(x)
  2D-3D8/1(y) -> fuzzy_logic_system7/4(w)
  3D-2D9/1(y) -> Integrator8/1
  fuzzy_adaptive_law9/1(wdot) -> 3D-2D9/1(x)
  Integrator8/1 -> 2D-3D9/1(x)
  2D-3D9/1(y) -> fuzzy_logic_system8/4(w)
  z2/1 -> fuzzy_adaptive_law4/5(w), fuzzy_adaptive_law5/5(w), fuzzy_adaptive_law6/5(w)
  z3/1 -> fuzzy_adaptive_law7/5(w), fuzzy_adaptive_law8/5(w), fuzzy_adaptive_law9/5(w)
  fuzzy_logic_system1/1(aF) -> Out1/1
  fuzzy_logic_system2/1(aF) -> Out2/1
  fuzzy_logic_system3/1(aF) -> Out3/1
  fuzzy_logic_system4/1(aF) -> Out4/1
  fuzzy_logic_system5/1(aF) -> Out5/1
  fuzzy_logic_system10/1(aF) -> Out6/1
  fuzzy_logic_system6/1(aF) -> aF/1
  fuzzy_logic_system7/1(aF) -> Out8/1
  fuzzy_logic_system8/1(aF) -> Out9/1
  w2/1 -> fuzzy_adaptive_law4/1(x1), fuzzy_adaptive_law7/1(x1), fuzzy_adaptive_law8/1(x1), fuzzy_adaptive_law9/1(x1), fuzzy_adaptive_law5/1(x1), fuzzy_adaptive_law6/1(x1)
  w1/1 -> fuzzy_adaptive_law1/5(w), fuzzy_adaptive_law3/1(x1), fuzzy_adaptive_law2/1(x1)

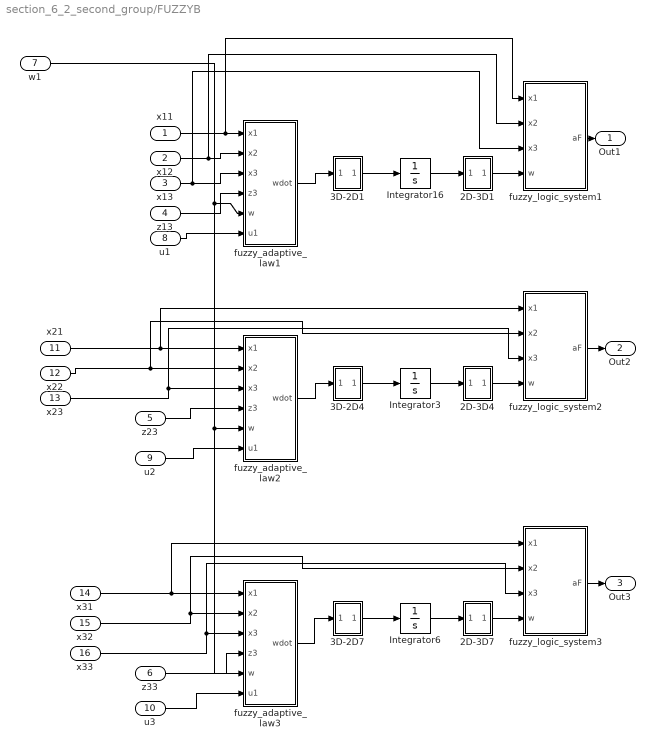
== system section_6_2_second_group/FUZZYB ==
  x11 : Inport
  x12 : Inport  Port=2
  x13 : Inport  Port=3
  z13 : Inport  Port=4
  z23 : Inport  Port=5
  z33 : Inport  Port=6
  w1 : Inport  Port=7
  u1 : Inport  Port=8
  u2 : Inport  Port=9
  u3 : Inport  Port=10
  x21 : Inport  Port=11
  x22 : Inport  Port=12
  x23 : Inport  Port=13
  x31 : Inport  Port=14
  x32 : Inport  Port=15
  x33 : Inport  Port=16
  2D-3D1 : MATLAB Function  TreatAsAtomicUnit=on
  2D-3D4 : MATLAB Function  TreatAsAtomicUnit=on
  2D-3D7 : MATLAB Function  TreatAsAtomicUnit=on
  3D-2D1 : MATLAB Function  TreatAsAtomicUnit=on
  3D-2D4 : MATLAB Function  TreatAsAtomicUnit=on
  3D-2D7 : MATLAB Function  TreatAsAtomicUnit=on
  Integrator16 : Integrator
  Integrator3 : Integrator
  Integrator6 : Integrator
  fuzzy_adaptive_law1 : MATLAB Function  TreatAsAtomicUnit=on
  fuzzy_adaptive_law2 : MATLAB Function  TreatAsAtomicUnit=on
  fuzzy_adaptive_law3 : MATLAB Function  TreatAsAtomicUnit=on
  fuzzy_logic_system1 : MATLAB Function  TreatAsAtomicUnit=on
  fuzzy_logic_system2 : MATLAB Function  TreatAsAtomicUnit=on
  fuzzy_logic_system3 : MATLAB Function  TreatAsAtomicUnit=on
  Out1 : Outport
  Out2 : Outport  Port=2
  Out3 : Outport  Port=3
  wires:
  3D-2D1/1(y) -> Integrator16/1
  fuzzy_adaptive_law1/1(wdot) -> 3D-2D1/1(x)
  Integrator16/1 -> 2D-3D1/1(x)
  2D-3D1/1(y) -> fuzzy_logic_system1/4(w)
  x11/1 -> fuzzy_logic_system1/1(x1), fuzzy_adaptive_law1/1(x1)
  x12/1 -> fuzzy_adaptive_law1/2(x2), fuzzy_logic_system1/2(x2)
  x13/1 -> fuzzy_adaptive_law1/3(x3), fuzzy_logic_system1/3(x3)
  z13/1 -> fuzzy_adaptive_law1/4(z3)
  3D-2D4/1(y) -> Integrator3/1
  fuzzy_adaptive_law2/1(wdot) -> 3D-2D4/1(x)
  Integrator3/1 -> 2D-3D4/1(x)
  2D-3D4/1(y) -> fuzzy_logic_system2/4(w)
  3D-2D7/1(y) -> Integrator6/1
  fuzzy_adaptive_law3/1(wdot) -> 3D-2D7/1(x)
  Integrator6/1 -> 2D-3D7/1(x)
  2D-3D7/1(y) -> fuzzy_logic_system3/4(w)
  fuzzy_logic_system1/1(aF) -> Out1/1
  fuzzy_logic_system2/1(aF) -> Out2/1
  fuzzy_logic_system3/1(aF) -> Out3/1
  w1/1 -> fuzzy_adaptive_law3/5(w), fuzzy_adaptive_law2/5(w), fuzzy_adaptive_law1/5(w)
  u1/1 -> fuzzy_adaptive_law1/6(u1)
  x23/1 -> fuzzy_adaptive_law2/3(x3), fuzzy_logic_system2/3(x3)
  x21/1 -> fuzzy_adaptive_law2/1(x1), fuzzy_logic_system2/1(x1)
  x31/1 -> fuzzy_adaptive_law3/1(x1), fuzzy_logic_system3/1(x1)
  x32/1 -> fuzzy_adaptive_law3/2(x2), fuzzy_logic_system3/2(x2)
  x33/1 -> fuzzy_adaptive_law3/3(x3), fuzzy_logic_system3/3(x3)
  x22/1 -> fuzzy_logic_system2/2(x2), fuzzy_adaptive_law2/2(x2)
  z23/1 -> fuzzy_adaptive_law2/4(z3)
  u2/1 -> fuzzy_adaptive_law2/6(u1)
  z33/1 -> fuzzy_adaptive_law3/4(z3)
  u3/1 -> fuzzy_adaptive_law3/6(u1)

== matlab function section_6_2_second_group/FUZZY3/fuzzy_adaptive_law3 ==
  data: wdot output; x1 input; x2 input; x3 input; zz input; w input
function wdot   = fcn(x1,x2,x3,zz,w)
delta=0.01;
ux1=zeros(5,1);
ux2=zeros(5,1);
ux3=zeros(5,1);
%%x1 5条模糊规则

z=zeros(5,6);
for j=1:5
    z(j,1)=-2+j-delta;
end
for j=6:10
    z(j-5,2)=-2+(j-5)-delta;
end
for j=11:15
    z(j-10,3)=-2+(j-10)-delta;
end

h1=1;%%规则间距
if x1<=-2-delta
    ux1(1,1)=1;
end

if x1>=-2-delta&&x1<=-1-delta
    ux1(1,1)=0.5*sin(pi*(x1-(-2-delta))/h1+0.5*pi)+0.5;
end

if x1>=-2-delta&&x1<=0-delta
    ux1(2,1)=0.5*sin(pi*(x1-(-1-delta))/h1+0.5*pi)+0.5;
end

if x1>=-1-delta&&x1<=1-delta
    ux1(3,1)=0.5*sin(pi*(x1-(0-delta))/h1+0.5*pi)+0.5;
end

if x1>=0-delta&&x1<=2-delta
    ux1(4,1)=0.5*sin(pi*(x1-(1-delta))/h1+0.5*pi)+0.5;
end

if x1>=1-delta&&x1<=2-delta
    ux1(5,1)=0.5*sin(pi*(x1-(2-delta))/h1+0.5*pi)+0.5;
end

if x1>2-delta
    ux1(5,1)=1;
end


h2=1;%%规则间距
if x2<=-2-delta
    ux2(1,1)=1;
end

if x2>=-2-delta&&x2<=-1-delta
    ux2(1,1)=0.5*sin(pi*(x2-(-2-delta))/h2+0.5*pi)+0.5;
end

if x2>=-2-delta&&x2<=0-delta
    ux2(2,1)=0.5*sin(pi*(x2-(-1-delta))/h2+0.5*pi)+0.5;
end

if x2>=-1-delta&&x2<=1-delta
    ux2(3,1)=0.5*sin(pi*(x2-(0-delta))/h2+0.5*pi)+0.5;
end

if x2>=0-delta&&x2<=2-delta
    ux2(4,1)=0.5*sin(pi*(x2-(1-delta))/h2+0.5*pi)+0.5;
end

if x2>=1-delta&&x2<=2-delta
    ux2(5,1)=0.5*sin(pi*(x2-(2-delta))/h2+0.5*pi)+0.5;
end

if x2>2-delta
    ux2(5,1)=1;
end

h3=1;%%规则间距
if x3<=-2-delta
    ux3(1,1)=1;
end

if x3>=-2-delta&&x3<=-1-delta
    ux3(1,1)=0.5*sin(pi*(x3-(-2-delta))/h3+0.5*pi)+0.5;
end

if x3>=-2-delta&&x3<=0-delta
    ux3(2,1)=0.5*sin(pi*(x3-(-1-delta))/h3+0.5*pi)+0.5;
end

if x3>=-1-delta&&x3<=1-delta
    ux3(3,1)=0.5*sin(pi*(x3-(0-delta))/h3+0.5*pi)+0.5;
end

if x3>=0-delta&&x3<=2-delta
    ux3(4,1)=0.5*sin(pi*(x3-(1-delta))/h3+0.5*pi)+0.5;
end

if x3>=1-delta&&x3<=2-delta
    ux3(5,1)=0.5*sin(pi*(x3-(2-delta))/h3+0.5*pi)+0.5;
end

if x3>2-delta
    ux3(5,1)=1;
end


%中心平均解模糊
Basic=0;
for i1=1:5
    for i2=1:5
        for i3=1:5
            Basic=Basic+ux1(i1,1)*ux2(i2,1)*ux3(i3,1);  
        end
    end
end

beta=zeros(5,5,5);
for i1=1:5
    for i2=1:5
        for i3=1:5
            beta(i1,i2,i3)=ux1(i1,1)*ux2(i2,1)*ux3(i3,1)/Basic;
        end
    end
end

wdot=zeros(5,5,5);
for i1=1:5
    for i2=1:5
        for i3=1:5
            wdot(i1,i2,i3)=w*beta(i1,i2,i3)*zz*z(i3,1);
        end
    end
end

end

== matlab function section_6_2_second_group/FUZZY3/fuzzy_adaptive_law4 ==
  data: wdot output; x1 input; x2 input; x3 input; zz input; w input
function wdot   = fcn(x1,x2,x3,zz,w)
delta=0.01;
ux1=zeros(5,1);
ux2=zeros(5,1);
ux3=zeros(5,1);
%%x1 5条模糊规则

z=zeros(5,6);
for j=1:5
    z(j,1)=-2+j-delta;
end
for j=6:10
    z(j-5,2)=-2+(j-5)-delta;
end
for j=11:15
    z(j-10,3)=-2+(j-10)-delta;
end

h1=1;%%规则间距
if x1<=-2-delta
    ux1(1,1)=1;
end

if x1>=-2-delta&&x1<=-1-delta
    ux1(1,1)=0.5*sin(pi*(x1-(-2-delta))/h1+0.5*pi)+0.5;
end

if x1>=-2-delta&&x1<=0-delta
    ux1(2,1)=0.5*sin(pi*(x1-(-1-delta))/h1+0.5*pi)+0.5;
end

if x1>=-1-delta&&x1<=1-delta
    ux1(3,1)=0.5*sin(pi*(x1-(0-delta))/h1+0.5*pi)+0.5;
end

if x1>=0-delta&&x1<=2-delta
    ux1(4,1)=0.5*sin(pi*(x1-(1-delta))/h1+0.5*pi)+0.5;
end

if x1>=1-delta&&x1<=2-delta
    ux1(5,1)=0.5*sin(pi*(x1-(2-delta))/h1+0.5*pi)+0.5;
end

if x1>2-delta
    ux1(5,1)=1;
end


h2=1;%%规则间距
if x2<=-2-delta
    ux2(1,1)=1;
end

if x2>=-2-delta&&x2<=-1-delta
    ux2(1,1)=0.5*sin(pi*(x2-(-2-delta))/h2+0.5*pi)+0.5;
end

if x2>=-2-delta&&x2<=0-delta
    ux2(2,1)=0.5*sin(pi*(x2-(-1-delta))/h2+0.5*pi)+0.5;
end

if x2>=-1-delta&&x2<=1-delta
    ux2(3,1)=0.5*sin(pi*(x2-(0-delta))/h2+0.5*pi)+0.5;
end

if x2>=0-delta&&x2<=2-delta
    ux2(4,1)=0.5*sin(pi*(x2-(1-delta))/h2+0.5*pi)+0.5;
end

if x2>=1-delta&&x2<=2-delta
    ux2(5,1)=0.5*sin(pi*(x2-(2-delta))/h2+0.5*pi)+0.5;
end

if x2>2-delta
    ux2(5,1)=1;
end

h3=1;%%规则间距
if x3<=-2-delta
    ux3(1,1)=1;
end

if x3>=-2-delta&&x3<=-1-delta
    ux3(1,1)=0.5*sin(pi*(x3-(-2-delta))/h3+0.5*pi)+0.5;
end

if x3>=-2-delta&&x3<=0-delta
    ux3(2,1)=0.5*sin(pi*(x3-(-1-delta))/h3+0.5*pi)+0.5;
end

if x3>=-1-delta&&x3<=1-delta
    ux3(3,1)=0.5*sin(pi*(x3-(0-delta))/h3+0.5*pi)+0.5;
end

if x3>=0-delta&&x3<=2-delta
    ux3(4,1)=0.5*sin(pi*(x3-(1-delta))/h3+0.5*pi)+0.5;
end

if x3>=1-delta&&x3<=2-delta
    ux3(5,1)=0.5*sin(pi*(x3-(2-delta))/h3+0.5*pi)+0.5;
end

if x3>2-delta
    ux3(5,1)=1;
end


%中心平均解模糊
Basic=0;
for i1=1:5
    for i2=1:5
        for i3=1:5
            Basic=Basic+ux1(i1,1)*ux2(i2,1)*ux3(i3,1);  
        end
    end
end

beta=zeros(5,5,5);
for i1=1:5
    for i2=1:5
        for i3=1:5
            beta(i1,i2,i3)=ux1(i1,1)*ux2(i2,1)*ux3(i3,1)/Basic;
        end
    end
end

wdot=zeros(5,5,5);
for i1=1:5
    for i2=1:5
        for i3=1:5
            wdot(i1,i2,i3)=w*beta(i1,i2,i3)*zz*z(i3,1);
        end
    end
end

end

== matlab function section_6_2_second_group/FUZZY3/fuzzy_adaptive_law5 ==
  data: wdot output; x1 input; x2 input; x3 input; zz input; w input
function wdot   = fcn(x1,x2,x3,zz,w)
delta=0.01;
ux1=zeros(5,1);
ux2=zeros(5,1);
ux3=zeros(5,1);
%%x1 5条模糊规则

z=zeros(5,6);
for j=1:5
    z(j,1)=-2+j-delta;
end
for j=6:10
    z(j-5,2)=-2+(j-5)-delta;
end
for j=11:15
    z(j-10,3)=-2+(j-10)-delta;
end

h1=1;%%规则间距
if x1<=-2-delta
    ux1(1,1)=1;
end

if x1>=-2-delta&&x1<=-1-delta
    ux1(1,1)=0.5*sin(pi*(x1-(-2-delta))/h1+0.5*pi)+0.5;
end

if x1>=-2-delta&&x1<=0-delta
    ux1(2,1)=0.5*sin(pi*(x1-(-1-delta))/h1+0.5*pi)+0.5;
end

if x1>=-1-delta&&x1<=1-delta
    ux1(3,1)=0.5*sin(pi*(x1-(0-delta))/h1+0.5*pi)+0.5;
end

if x1>=0-delta&&x1<=2-delta
    ux1(4,1)=0.5*sin(pi*(x1-(1-delta))/h1+0.5*pi)+0.5;
end

if x1>=1-delta&&x1<=2-delta
    ux1(5,1)=0.5*sin(pi*(x1-(2-delta))/h1+0.5*pi)+0.5;
end

if x1>2-delta
    ux1(5,1)=1;
end


h2=1;%%规则间距
if x2<=-2-delta
    ux2(1,1)=1;
end

if x2>=-2-delta&&x2<=-1-delta
    ux2(1,1)=0.5*sin(pi*(x2-(-2-delta))/h2+0.5*pi)+0.5;
end

if x2>=-2-delta&&x2<=0-delta
    ux2(2,1)=0.5*sin(pi*(x2-(-1-delta))/h2+0.5*pi)+0.5;
end

if x2>=-1-delta&&x2<=1-delta
    ux2(3,1)=0.5*sin(pi*(x2-(0-delta))/h2+0.5*pi)+0.5;
end

if x2>=0-delta&&x2<=2-delta
    ux2(4,1)=0.5*sin(pi*(x2-(1-delta))/h2+0.5*pi)+0.5;
end

if x2>=1-delta&&x2<=2-delta
    ux2(5,1)=0.5*sin(pi*(x2-(2-delta))/h2+0.5*pi)+0.5;
end

if x2>2-delta
    ux2(5,1)=1;
end

h3=1;%%规则间距
if x3<=-2-delta
    ux3(1,1)=1;
end

if x3>=-2-delta&&x3<=-1-delta
    ux3(1,1)=0.5*sin(pi*(x3-(-2-delta))/h3+0.5*pi)+0.5;
end

if x3>=-2-delta&&x3<=0-delta
    ux3(2,1)=0.5*sin(pi*(x3-(-1-delta))/h3+0.5*pi)+0.5;
end

if x3>=-1-delta&&x3<=1-delta
    ux3(3,1)=0.5*sin(pi*(x3-(0-delta))/h3+0.5*pi)+0.5;
end

if x3>=0-delta&&x3<=2-delta
    ux3(4,1)=0.5*sin(pi*(x3-(1-delta))/h3+0.5*pi)+0.5;
end

if x3>=1-delta&&x3<=2-delta
    ux3(5,1)=0.5*sin(pi*(x3-(2-delta))/h3+0.5*pi)+0.5;
end

if x3>2-delta
    ux3(5,1)=1;
end


%中心平均解模糊
Basic=0;
for i1=1:5
    for i2=1:5
        for i3=1:5
            Basic=Basic+ux1(i1,1)*ux2(i2,1)*ux3(i3,1);  
        end
    end
end

beta=zeros(5,5,5);
for i1=1:5
    for i2=1:5
        for i3=1:5
            beta(i1,i2,i3)=ux1(i1,1)*ux2(i2,1)*ux3(i3,1)/Basic;
        end
    end
end

wdot=zeros(5,5,5);
for i1=1:5
    for i2=1:5
        for i3=1:5
            wdot(i1,i2,i3)=w*beta(i1,i2,i3)*zz*z(i3,1);
        end
    end
end

end

== matlab function section_6_2_second_group/FUZZY3/fuzzy_adaptive_law6 ==
  data: wdot output; x1 input; x2 input; x3 input; zz input; w input
function wdot   = fcn(x1,x2,x3,zz,w)
delta=0.01;
ux1=zeros(5,1);
ux2=zeros(5,1);
ux3=zeros(5,1);
%%x1 5条模糊规则

z=zeros(5,6);
for j=1:5
    z(j,1)=-2+j-delta;
end
for j=6:10
    z(j-5,2)=-2+(j-5)-delta;
end
for j=11:15
    z(j-10,3)=-2+(j-10)-delta;
end

h1=1;%%规则间距
if x1<=-2-delta
    ux1(1,1)=1;
end

if x1>=-2-delta&&x1<=-1-delta
    ux1(1,1)=0.5*sin(pi*(x1-(-2-delta))/h1+0.5*pi)+0.5;
end

if x1>=-2-delta&&x1<=0-delta
    ux1(2,1)=0.5*sin(pi*(x1-(-1-delta))/h1+0.5*pi)+0.5;
end

if x1>=-1-delta&&x1<=1-delta
    ux1(3,1)=0.5*sin(pi*(x1-(0-delta))/h1+0.5*pi)+0.5;
end

if x1>=0-delta&&x1<=2-delta
    ux1(4,1)=0.5*sin(pi*(x1-(1-delta))/h1+0.5*pi)+0.5;
end

if x1>=1-delta&&x1<=2-delta
    ux1(5,1)=0.5*sin(pi*(x1-(2-delta))/h1+0.5*pi)+0.5;
end

if x1>2-delta
    ux1(5,1)=1;
end


h2=1;%%规则间距
if x2<=-2-delta
    ux2(1,1)=1;
end

if x2>=-2-delta&&x2<=-1-delta
    ux2(1,1)=0.5*sin(pi*(x2-(-2-delta))/h2+0.5*pi)+0.5;
end

if x2>=-2-delta&&x2<=0-delta
    ux2(2,1)=0.5*sin(pi*(x2-(-1-delta))/h2+0.5*pi)+0.5;
end

if x2>=-1-delta&&x2<=1-delta
    ux2(3,1)=0.5*sin(pi*(x2-(0-delta))/h2+0.5*pi)+0.5;
end

if x2>=0-delta&&x2<=2-delta
    ux2(4,1)=0.5*sin(pi*(x2-(1-delta))/h2+0.5*pi)+0.5;
end

if x2>=1-delta&&x2<=2-delta
    ux2(5,1)=0.5*sin(pi*(x2-(2-delta))/h2+0.5*pi)+0.5;
end

if x2>2-delta
    ux2(5,1)=1;
end

h3=1;%%规则间距
if x3<=-2-delta
    ux3(1,1)=1;
end

if x3>=-2-delta&&x3<=-1-delta
    ux3(1,1)=0.5*sin(pi*(x3-(-2-delta))/h3+0.5*pi)+0.5;
end

if x3>=-2-delta&&x3<=0-delta
    ux3(2,1)=0.5*sin(pi*(x3-(-1-delta))/h3+0.5*pi)+0.5;
end

if x3>=-1-delta&&x3<=1-delta
    ux3(3,1)=0.5*sin(pi*(x3-(0-delta))/h3+0.5*pi)+0.5;
end

if x3>=0-delta&&x3<=2-delta
    ux3(4,1)=0.5*sin(pi*(x3-(1-delta))/h3+0.5*pi)+0.5;
end

if x3>=1-delta&&x3<=2-delta
    ux3(5,1)=0.5*sin(pi*(x3-(2-delta))/h3+0.5*pi)+0.5;
end

if x3>2-delta
    ux3(5,1)=1;
end


%中心平均解模糊
Basic=0;
for i1=1:5
    for i2=1:5
        for i3=1:5
            Basic=Basic+ux1(i1,1)*ux2(i2,1)*ux3(i3,1);  
        end
    end
end

beta=zeros(5,5,5);
for i1=1:5
    for i2=1:5
        for i3=1:5
            beta(i1,i2,i3)=ux1(i1,1)*ux2(i2,1)*ux3(i3,1)/Basic;
        end
    end
end

wdot=zeros(5,5,5);
for i1=1:5
    for i2=1:5
        for i3=1:5
            wdot(i1,i2,i3)=w*beta(i1,i2,i3)*zz*z(i3,1);
        end
    end
end

end

== matlab function section_6_2_second_group/FUZZY3/fuzzy_adaptive_law7 ==
  data: wdot output; x1 input; x2 input; x3 input; zz input; w input
function wdot   = fcn(x1,x2,x3,zz,w)
delta=0.01;
ux1=zeros(5,1);
ux2=zeros(5,1);
ux3=zeros(5,1);
%%x1 5条模糊规则

z=zeros(5,6);
for j=1:5
    z(j,1)=-2+j-delta;
end
for j=6:10
    z(j-5,2)=-2+(j-5)-delta;
end
for j=11:15
    z(j-10,3)=-2+(j-10)-delta;
end

h1=1;%%规则间距
if x1<=-2-delta
    ux1(1,1)=1;
end

if x1>=-2-delta&&x1<=-1-delta
    ux1(1,1)=0.5*sin(pi*(x1-(-2-delta))/h1+0.5*pi)+0.5;
end

if x1>=-2-delta&&x1<=0-delta
    ux1(2,1)=0.5*sin(pi*(x1-(-1-delta))/h1+0.5*pi)+0.5;
end

if x1>=-1-delta&&x1<=1-delta
    ux1(3,1)=0.5*sin(pi*(x1-(0-delta))/h1+0.5*pi)+0.5;
end

if x1>=0-delta&&x1<=2-delta
    ux1(4,1)=0.5*sin(pi*(x1-(1-delta))/h1+0.5*pi)+0.5;
end

if x1>=1-delta&&x1<=2-delta
    ux1(5,1)=0.5*sin(pi*(x1-(2-delta))/h1+0.5*pi)+0.5;
end

if x1>2-delta
    ux1(5,1)=1;
end


h2=1;%%规则间距
if x2<=-2-delta
    ux2(1,1)=1;
end

if x2>=-2-delta&&x2<=-1-delta
    ux2(1,1)=0.5*sin(pi*(x2-(-2-delta))/h2+0.5*pi)+0.5;
end

if x2>=-2-delta&&x2<=0-delta
    ux2(2,1)=0.5*sin(pi*(x2-(-1-delta))/h2+0.5*pi)+0.5;
end

if x2>=-1-delta&&x2<=1-delta
    ux2(3,1)=0.5*sin(pi*(x2-(0-delta))/h2+0.5*pi)+0.5;
end

if x2>=0-delta&&x2<=2-delta
    ux2(4,1)=0.5*sin(pi*(x2-(1-delta))/h2+0.5*pi)+0.5;
end

if x2>=1-delta&&x2<=2-delta
    ux2(5,1)=0.5*sin(pi*(x2-(2-delta))/h2+0.5*pi)+0.5;
end

if x2>2-delta
    ux2(5,1)=1;
end

h3=1;%%规则间距
if x3<=-2-delta
    ux3(1,1)=1;
end

if x3>=-2-delta&&x3<=-1-delta
    ux3(1,1)=0.5*sin(pi*(x3-(-2-delta))/h3+0.5*pi)+0.5;
end

if x3>=-2-delta&&x3<=0-delta
    ux3(2,1)=0.5*sin(pi*(x3-(-1-delta))/h3+0.5*pi)+0.5;
end

if x3>=-1-delta&&x3<=1-delta
    ux3(3,1)=0.5*sin(pi*(x3-(0-delta))/h3+0.5*pi)+0.5;
end

if x3>=0-delta&&x3<=2-delta
    ux3(4,1)=0.5*sin(pi*(x3-(1-delta))/h3+0.5*pi)+0.5;
end

if x3>=1-delta&&x3<=2-delta
    ux3(5,1)=0.5*sin(pi*(x3-(2-delta))/h3+0.5*pi)+0.5;
end

if x3>2-delta
    ux3(5,1)=1;
end


%中心平均解模糊
Basic=0;
for i1=1:5
    for i2=1:5
        for i3=1:5
            Basic=Basic+ux1(i1,1)*ux2(i2,1)*ux3(i3,1);  
        end
    end
end

beta=zeros(5,5,5);
for i1=1:5
    for i2=1:5
        for i3=1:5
            beta(i1,i2,i3)=ux1(i1,1)*ux2(i2,1)*ux3(i3,1)/Basic;
        end
    end
end

wdot=zeros(5,5,5);
for i1=1:5
    for i2=1:5
        for i3=1:5
            wdot(i1,i2,i3)=w*beta(i1,i2,i3)*zz*z(i3,1);
        end
    end
end

end

== matlab function section_6_2_second_group/FUZZY3/fuzzy_adaptive_law8 ==
  data: wdot output; x1 input; x2 input; x3 input; zz input; w input
function wdot   = fcn(x1,x2,x3,zz,w)
delta=0.01;
ux1=zeros(5,1);
ux2=zeros(5,1);
ux3=zeros(5,1);
%%x1 5条模糊规则

z=zeros(5,6);
for j=1:5
    z(j,1)=-2+j-delta;
end
for j=6:10
    z(j-5,2)=-2+(j-5)-delta;
end
for j=11:15
    z(j-10,3)=-2+(j-10)-delta;
end

h1=1;%%规则间距
if x1<=-2-delta
    ux1(1,1)=1;
end

if x1>=-2-delta&&x1<=-1-delta
    ux1(1,1)=0.5*sin(pi*(x1-(-2-delta))/h1+0.5*pi)+0.5;
end

if x1>=-2-delta&&x1<=0-delta
    ux1(2,1)=0.5*sin(pi*(x1-(-1-delta))/h1+0.5*pi)+0.5;
end

if x1>=-1-delta&&x1<=1-delta
    ux1(3,1)=0.5*sin(pi*(x1-(0-delta))/h1+0.5*pi)+0.5;
end

if x1>=0-delta&&x1<=2-delta
    ux1(4,1)=0.5*sin(pi*(x1-(1-delta))/h1+0.5*pi)+0.5;
end

if x1>=1-delta&&x1<=2-delta
    ux1(5,1)=0.5*sin(pi*(x1-(2-delta))/h1+0.5*pi)+0.5;
end

if x1>2-delta
    ux1(5,1)=1;
end


h2=1;%%规则间距
if x2<=-2-delta
    ux2(1,1)=1;
end

if x2>=-2-delta&&x2<=-1-delta
    ux2(1,1)=0.5*sin(pi*(x2-(-2-delta))/h2+0.5*pi)+0.5;
end

if x2>=-2-delta&&x2<=0-delta
    ux2(2,1)=0.5*sin(pi*(x2-(-1-delta))/h2+0.5*pi)+0.5;
end

if x2>=-1-delta&&x2<=1-delta
    ux2(3,1)=0.5*sin(pi*(x2-(0-delta))/h2+0.5*pi)+0.5;
end

if x2>=0-delta&&x2<=2-delta
    ux2(4,1)=0.5*sin(pi*(x2-(1-delta))/h2+0.5*pi)+0.5;
end

if x2>=1-delta&&x2<=2-delta
    ux2(5,1)=0.5*sin(pi*(x2-(2-delta))/h2+0.5*pi)+0.5;
end

if x2>2-delta
    ux2(5,1)=1;
end

h3=1;%%规则间距
if x3<=-2-delta
    ux3(1,1)=1;
end

if x3>=-2-delta&&x3<=-1-delta
    ux3(1,1)=0.5*sin(pi*(x3-(-2-delta))/h3+0.5*pi)+0.5;
end

if x3>=-2-delta&&x3<=0-delta
    ux3(2,1)=0.5*sin(pi*(x3-(-1-delta))/h3+0.5*pi)+0.5;
end

if x3>=-1-delta&&x3<=1-delta
    ux3(3,1)=0.5*sin(pi*(x3-(0-delta))/h3+0.5*pi)+0.5;
end

if x3>=0-delta&&x3<=2-delta
    ux3(4,1)=0.5*sin(pi*(x3-(1-delta))/h3+0.5*pi)+0.5;
end

if x3>=1-delta&&x3<=2-delta
    ux3(5,1)=0.5*sin(pi*(x3-(2-delta))/h3+0.5*pi)+0.5;
end

if x3>2-delta
    ux3(5,1)=1;
end


%中心平均解模糊
Basic=0;
for i1=1:5
    for i2=1:5
        for i3=1:5
            Basic=Basic+ux1(i1,1)*ux2(i2,1)*ux3(i3,1);  
        end
    end
end

beta=zeros(5,5,5);
for i1=1:5
    for i2=1:5
        for i3=1:5
            beta(i1,i2,i3)=ux1(i1,1)*ux2(i2,1)*ux3(i3,1)/Basic;
        end
    end
end

wdot=zeros(5,5,5);
for i1=1:5
    for i2=1:5
        for i3=1:5
            wdot(i1,i2,i3)=w*beta(i1,i2,i3)*zz*z(i3,1);
        end
    end
end

end

== matlab function section_6_2_second_group/FUZZY3/fuzzy_adaptive_law9 ==
  data: wdot output; x1 input; x2 input; x3 input; zz input; w input
function wdot   = fcn(x1,x2,x3,zz,w)
delta=0.01;
ux1=zeros(5,1);
ux2=zeros(5,1);
ux3=zeros(5,1);
%%x1 5条模糊规则

z=zeros(5,6);
for j=1:5
    z(j,1)=-2+j-delta;
end
for j=6:10
    z(j-5,2)=-2+(j-5)-delta;
end
for j=11:15
    z(j-10,3)=-2+(j-10)-delta;
end

h1=1;%%规则间距
if x1<=-2-delta
    ux1(1,1)=1;
end

if x1>=-2-delta&&x1<=-1-delta
    ux1(1,1)=0.5*sin(pi*(x1-(-2-delta))/h1+0.5*pi)+0.5;
end

if x1>=-2-delta&&x1<=0-delta
    ux1(2,1)=0.5*sin(pi*(x1-(-1-delta))/h1+0.5*pi)+0.5;
end

if x1>=-1-delta&&x1<=1-delta
    ux1(3,1)=0.5*sin(pi*(x1-(0-delta))/h1+0.5*pi)+0.5;
end

if x1>=0-delta&&x1<=2-delta
    ux1(4,1)=0.5*sin(pi*(x1-(1-delta))/h1+0.5*pi)+0.5;
end

if x1>=1-delta&&x1<=2-delta
    ux1(5,1)=0.5*sin(pi*(x1-(2-delta))/h1+0.5*pi)+0.5;
end

if x1>2-delta
    ux1(5,1)=1;
end


h2=1;%%规则间距
if x2<=-2-delta
    ux2(1,1)=1;
end

if x2>=-2-delta&&x2<=-1-delta
    ux2(1,1)=0.5*sin(pi*(x2-(-2-delta))/h2+0.5*pi)+0.5;
end

if x2>=-2-delta&&x2<=0-delta
    ux2(2,1)=0.5*sin(pi*(x2-(-1-delta))/h2+0.5*pi)+0.5;
end

if x2>=-1-delta&&x2<=1-delta
    ux2(3,1)=0.5*sin(pi*(x2-(0-delta))/h2+0.5*pi)+0.5;
end

if x2>=0-delta&&x2<=2-delta
    ux2(4,1)=0.5*sin(pi*(x2-(1-delta))/h2+0.5*pi)+0.5;
end

if x2>=1-delta&&x2<=2-delta
    ux2(5,1)=0.5*sin(pi*(x2-(2-delta))/h2+0.5*pi)+0.5;
end

if x2>2-delta
    ux2(5,1)=1;
end

h3=1;%%规则间距
if x3<=-2-delta
    ux3(1,1)=1;
end

if x3>=-2-delta&&x3<=-1-delta
    ux3(1,1)=0.5*sin(pi*(x3-(-2-delta))/h3+0.5*pi)+0.5;
end

if x3>=-2-delta&&x3<=0-delta
    ux3(2,1)=0.5*sin(pi*(x3-(-1-delta))/h3+0.5*pi)+0.5;
end

if x3>=-1-delta&&x3<=1-delta
    ux3(3,1)=0.5*sin(pi*(x3-(0-delta))/h3+0.5*pi)+0.5;
end

if x3>=0-delta&&x3<=2-delta
    ux3(4,1)=0.5*sin(pi*(x3-(1-delta))/h3+0.5*pi)+0.5;
end

if x3>=1-delta&&x3<=2-delta
    ux3(5,1)=0.5*sin(pi*(x3-(2-delta))/h3+0.5*pi)+0.5;
end

if x3>2-delta
    ux3(5,1)=1;
end


%中心平均解模糊
Basic=0;
for i1=1:5
    for i2=1:5
        for i3=1:5
            Basic=Basic+ux1(i1,1)*ux2(i2,1)*ux3(i3,1);  
        end
    end
end

beta=zeros(5,5,5);
for i1=1:5
    for i2=1:5
        for i3=1:5
            beta(i1,i2,i3)=ux1(i1,1)*ux2(i2,1)*ux3(i3,1)/Basic;
        end
    end
end

wdot=zeros(5,5,5);
for i1=1:5
    for i2=1:5
        for i3=1:5
            wdot(i1,i2,i3)=w*beta(i1,i2,i3)*zz*z(i3,1);
        end
    end
end

end
